simulink model "NDI"  (R2021a)
settings: Solver=VariableStepAuto  StartTime=0.0  StopTime=30  MaxStep=0.0001  RelTol=1e-3
undefined symbols (not defined in the file): K3, N3, q01, q02, tau0
settings Model: Creator=y.briere  LastModifiedBy=y.briere

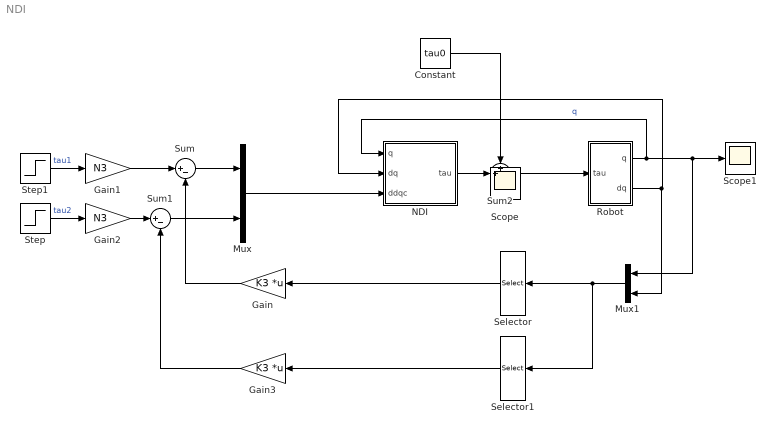
== system NDI ==
  Constant : Constant  Value=tau0
  Gain : Gain  Gain=K3  Multiplication=Matrix(K*u)
  Gain1 : Gain  Gain=N3
  Gain2 : Gain  Gain=N3
  Gain3 : Gain  Gain=K3  Multiplication=Matrix(K*u)
  Mux : Mux  Inputs=2
  Mux1 : Mux  Inputs=2
  NDI : Subsystem
  Robot : Subsystem
  Scope1 : Scope
  Selector : Selector  InputPortWidth=4  IndexOptions=Index vector (dialog)  Indices=[1 3]  OutputSizes=1
  Selector1 : Selector  InputPortWidth=4  IndexOptions=Index vector (dialog)  Indices=[2 4]  OutputSizes=1
  Step : Step  Time=10  Before=q02  After=q02  SampleTime=0
  Step1 : Step  Before=q01  After=q01+0.1  SampleTime=0
  Sum : Sum  Inputs=|+-
  Sum1 : Sum  Inputs=|+-
  Sum2 : Sum  Inputs=++|
  Scope : Scope
  wires:
  Sum1/1 -> Mux/2
  Sum/1 -> Mux/1
  Robot/1(q) -> NDI/1(q), Mux1/1, Scope1/1  "q"
  Selector/1 -> Gain/1
  Step1/1 -> Gain1/1  "tau1"
  Step/1 -> Gain2/1  "tau2"
  Gain2/1 -> Sum1/1
  Selector1/1 -> Gain3/1
  Gain/1 -> Sum/2
  Gain3/1 -> Sum1/2
  Mux1/1 -> Selector1/1, Selector/1
  Gain1/1 -> Sum/1
  Sum2/1 -> Robot/1(tau)
  NDI/1(tau) -> Sum2/2
  Robot/2(dq) -> Mux1/2, NDI/2(dq)
  Mux/1 -> NDI/3(ddqc)
  Constant/1 -> Sum2/1

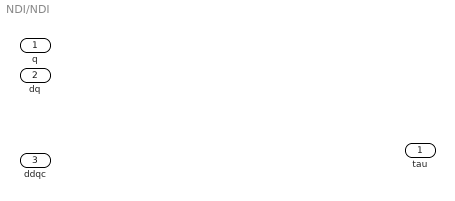
== system NDI/NDI ==
  q : Inport
  dq : Inport  Port=2
  ddqc : Inport  Port=3
  tau : Outport

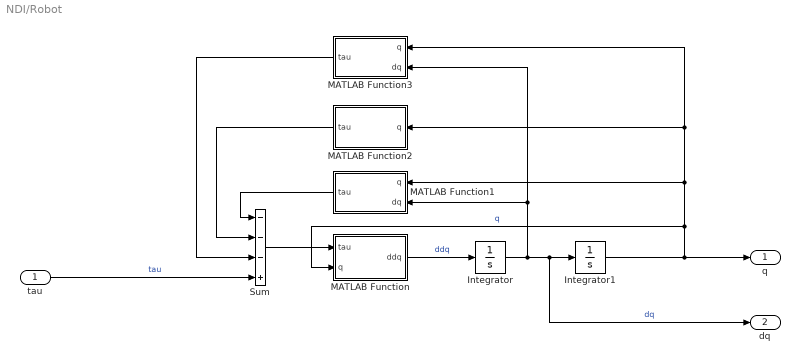
== system NDI/Robot ==
  tau : Inport
  Integrator : Integrator  InitialCondition=[0:0]
  Integrator1 : Integrator  InitialCondition=[q01;q02]
  MATLAB Function : MATLAB Function  TreatAsAtomicUnit=on
  MATLAB Function1 : MATLAB Function  TreatAsAtomicUnit=on
  MATLAB Function2 : MATLAB Function  TreatAsAtomicUnit=on
  MATLAB Function3 : MATLAB Function  TreatAsAtomicUnit=on
  Sum : Sum  Inputs=---+
  q : Outport
  dq : Outport  Port=2
  wires:
  Integrator/1 -> MATLAB Function3/2(dq), MATLAB Function1/2(dq), dq/1, Integrator1/1  "dq"
  Integrator1/1 -> MATLAB Function3/1(q), MATLAB Function2/1(q), MATLAB Function1/1(q), MATLAB Function/2(q), q/1  "q"
  MATLAB Function3/1(tau) -> Sum/3
  MATLAB Function/1(ddq) -> Integrator/1  "ddq"
  Sum/1 -> MATLAB Function/1(tau)
  MATLAB Function1/1(tau) -> Sum/1
  MATLAB Function2/1(tau) -> Sum/2
  tau/1 -> Sum/4  "tau"

== matlab function NDI/Robot/MATLAB Function ==
  data: tau input; q input; ddq output
function ddq  = invM(tau,q)
% Mass matrix
R.m1 = 1; % Arm 1 mass
R.m2 = 1; % Arm 2 mass
R.L1 = 1; % Arm 1 length
R.L2 = 1; % Arm 2 length
M = [(R.m1*R.L1^2)/4+R.m2*(R.L1^2+R.L2^2/4+R.L1*R.L2*cos(q(2))) ,  R.m2*R.L2*(R.L2+ 2*R.L1*cos(q(2)))/4
    R.m2*R.L2*(R.L2+ 2*R.L1*cos(q(2)))/4                       ,  R.m2*R.L2^2/4];

ddq = M\tau;

== matlab function NDI/Robot/MATLAB Function1 ==
  data: q input; dq input; tau output
function tau  = coriolis(q,dq)
% Convective Matrix
%Robot parameters
R.m1 = 1; % Arm 1 mass
R.m2 = 1; % Arm 2 mass
R.L1 = 1; % Arm 1 length
R.L2 = 1; % Arm 2 length
Cm = [-R.m2*R.L1*R.L2*sin(q(2))*dq(2) -R.m2*R.L1*R.L2*sin(q(2))/2*dq(2);...
    R.m2*R.L1*R.L2*dq(1)*sin(q(2))/2 0];
tau = Cm*dq;

== matlab function NDI/Robot/MATLAB Function2 ==
  data: q input; tau output
function tau  = gravity(q)
%Robot parameters
R.m1 = 1; % Arm 1 mass
R.m2 = 1; % Arm 2 mass
R.L1 = 1; % Arm 1 length
R.L2 = 1; % Arm 2 length
R.g = 0*9.81; % Gravity

tau = [R.m1*R.g*R.L1*cos(q(1))/2+R.m2*R.g*(R.L2*cos(q(1)+q(2))/2+R.L1*cos(q(1)));...
    R.m2*R.g*R.L2*cos(q(1)+q(2))/2];

== matlab function NDI/Robot/MATLAB Function3 ==
  data: q input; dq input; tau output
function tau  = friction(q,dq)
%Robot parameters
R.f1 = 1; % Friction 1
R.f2 = 1; % Friction 2

tau = [R.f1
    R.f2].*dq;
